simulink model "chap10_1sim"  (Simulink 3.00)
settings: Solver=ode45  SolverMode=SingleTasking  StartTime=0.0  StopTime=3  FixedStep=0.001  RelTol=1e-3
settings Model: LastModifiedBy=liu

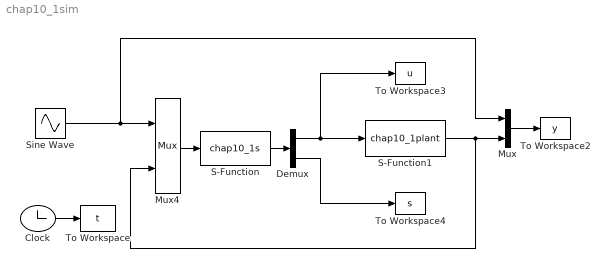
== system chap10_1sim ==
  Clock : Clock
  Demux : Demux  Outputs=2
  Mux : Mux  Inputs=2
  Mux4 : Mux  Inputs=2
      settings: DisplayOption=none
  S-Function : S-Function  FunctionName=chap10_1s  PortCounts=[]  SFunctionModules=''
  S-Function1 : S-Function  FunctionName=chap10_1plant  PortCounts=[]  SFunctionModules=''
  Sine Wave : Sin  Amplitude=0.5  Frequency=2*pi  Phase=0  SampleTime=0
  To Workspace : ToWorkspace  VariableName=t  SampleTime=-1  SaveFormat=Matrix
  To Workspace2 : ToWorkspace  VariableName=y  SampleTime=-1  SaveFormat=Matrix
  To Workspace3 : ToWorkspace  VariableName=u  SampleTime=-1  SaveFormat=Matrix
  To Workspace4 : ToWorkspace  VariableName=s  SampleTime=-1  SaveFormat=Matrix
  wires:
  Mux4/1 -> S-Function/1
  Clock/1 -> To Workspace/1
  Sine Wave/1 -> Mux/1, Mux4/1
  S-Function/1 -> Demux/1
  S-Function1/1 -> Mux4/2, Mux/2
  Mux/1 -> To Workspace2/1
  Demux/1 -> S-Function1/1, To Workspace3/1
  Demux/2 -> To Workspace4/1
